simulink model "TL"  (R2023a)
settings: Solver=VariableStepAuto  StartTime=0.0  StopTime=10.0  RelTol=1e-3
settings Model: Creator=13524  LastModifiedBy=13524

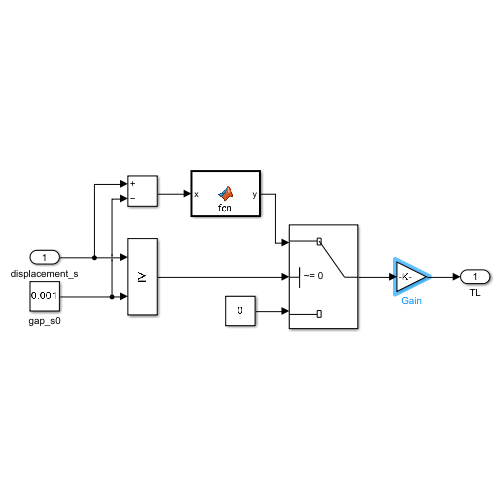
[thumbnail: Simulink's stored preview of the top-level diagram]
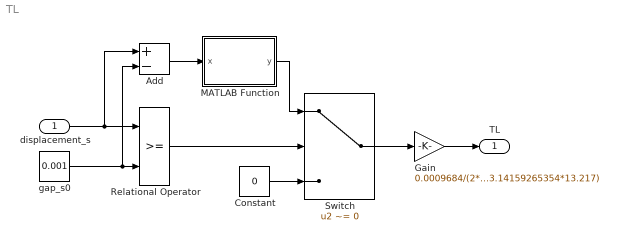
== system TL ==
  displacement_s : Inport
  Add : Sum  Inputs=+-
  Constant : Constant  Value=0
  Gain : Gain  Gain=0.0009684/(2*3.14159265354*13.217)
  MATLAB Function : MATLAB Function  TreatAsAtomicUnit=on
  Relational Operator : RelationalOperator  OutDataTypeStr=boolean  RndMeth=Simplest  InputSameDT=off
  Switch : Switch  Criteria=u2 ~= 0  ZeroCross=off  SaturateOnIntegerOverflow=off  InputSameDT=off
  gap_s0 : Constant  Value=0.001  VectorParams1D=off
  TL : Outport
  wires:
  displacement_s/1 -> Relational Operator/1, Add/1
  gap_s0/1 -> Add/2, Relational Operator/2
  Relational Operator/1 -> Switch/2
  Add/1 -> MATLAB Function/1(x)
  MATLAB Function/1(y) -> Switch/1
  Constant/1 -> Switch/3
  Switch/1 -> Gain/1
  Gain/1 -> TL/1

== matlab function TL/MATLAB Function ==
  data: x input; y output
function y = fcn(x)

y=-1917.2*x^3+29512*x^2-10223*x+959.33;
